simulink model "AGTF30SysDyn_PExPIn"  (R2023b)
settings: Solver=ode4  StartTime=0.0  StopTime=MWS.In.tend  FixedStep=MWS.In.Ts  RelTol=1e-3  EnableMultiTasking=on
model workspace: external: MAT-File (data not in the file)
values from neighbouring files (symbols this model uses):
  MWS = setup_initialize(MWS,startPt,SSsolverSP)    [Setup_Simulation.m]    (also in run_AGTF30e_script.m = Setup_Simulation(inputMethod,MWS.In,filename,Mdl,SSsolverSP))
undefined symbols (not defined in the file or in its folder): DiscIntNeverNeededParam
libraries: simulink x32, Lib_Solve_ModelSource_TMATS x28, Lib_EMTAT x27, Lib_Cntrl_FirstOrderSensor_TMATS x19, Lib_Cntrl_FirstOrderActuator_TMATS x2, Lib_Cntrl_LimitSelect_TMATS x2, Lib_Solve_OuterLoopIntegrator_TMATS x2, Lib_Cntrl_CorrectedSpeed_TMATS x1, Lib_Solve_IterNRSolverJC_TMATS x1, slpidlib x1
(part 5 of 8)

== system AGTF30SysDyn_PExPIn/Control System/Wf Controller/Controller/Wf Limit Controllers/Accel Controller ==
  Alt : Inport
  MN : Inport  Port=2
  N1cN : Inport  Port=3
  phiEPT : Inport  Port=4
  phiBoost : Inport  Port=5
  Wfmax : Inport  Port=6
  Wfcmd : Inport  Port=7
  ps3 : Inport  Port=8
  Constant : Constant  Value=MWS.In.Options.WfTransientLogic
  Constant1 : Constant  Value=MWS.In.Options.HybridConfig
  Constant10 : Constant  Value=MWS.In.Options.HybridConfig
  Constant11 : Constant  Value=1.0425
  Constant2 : Constant
  Constant3 : Constant  Value=-4*MWS.In.Ts
  Constant4 : Constant  Value=MWS.In.Options.TEEM
  Constant5 : Constant
  Constant6 : Constant  Value=1.068
  Constant7 : Constant  Value=1.04
  Constant8 : Constant  Value=MWS.In.Options.EngineEMInt
  Constant9 : Constant  Value=1.06
  Divide1 : Product  Inputs=**
  Divide2 : Product  Inputs=**
  Divide3 : Product  Inputs=*/
  Divide4 : Product  Inputs=**
  Gain2 : Gain  Gain=MWS.Cntrl.WfCntrl.GenAccel.CeilingMultiplier
  Math Function : Math
  Memory : Memory  InitialCondition=MWS.Init.IC.Wf
  Multiport Switch : MultiPortSwitch  SaturateOnIntegerOverflow=off  InputSameDT=off
  Multiport Switch1 : MultiPortSwitch  SaturateOnIntegerOverflow=off  InputSameDT=off
  RUSched_Boost : Lookup_n-D  NumberOfTableDimensions=5  BreakpointsForDimension1=MWS.Cntrl.WfCntrl.Accel.Boost.RUsch.N1cN_vec  BreakpointsForDimension2=MWS.Cntrl.WfCntrl.Accel.Boost.RUsch.Alt_vec  BreakpointsForDimension3=MWS.Cntrl.WfCntrl.Accel.Boost.RUsch.MN_vec  BreakpointsForDimension4=MWS.Cntrl.WfCntrl.Accel.Boost.RUsch.phiEPT_vec  BreakpointsForDimension5=MWS.Cntrl.WfCntrl.Accel.Boost.RUsch.phiBoost_vec  Table=MWS.Cntrl.WfCntrl.Accel.Boost.RUsch.RU_array  ExtrapMethod=Clip  InternalRulePriority=Speed  RndMeth=Simplest
      settings: InputPortMap=u0,u1,u2,u3,u4
  RUSched_PEx : Lookup_n-D  NumberOfTableDimensions=4  BreakpointsForDimension1=MWS.Cntrl.WfCntrl.Accel.PEx.RUsch.N1cN_vec  BreakpointsForDimension2=MWS.Cntrl.WfCntrl.Accel.PEx.RUsch.Alt_vec  BreakpointsForDimension3=MWS.Cntrl.WfCntrl.Accel.PEx.RUsch.MN_vec  BreakpointsForDimension4=MWS.Cntrl.WfCntrl.Accel.PEx.RUsch.phiEPT_vec  Table=MWS.Cntrl.WfCntrl.Accel.PEx.RUsch.RU_array  ExtrapMethod=Clip  InternalRulePriority=Speed  RndMeth=Simplest
      settings: InputPortMap=u0,u1,u2,u3
  RUSched_STD : Lookup_n-D  NumberOfTableDimensions=4  BreakpointsForDimension1=MWS.Cntrl.WfCntrl.Accel.STD.RUsch.N1cN_vec  BreakpointsForDimension2=MWS.Cntrl.WfCntrl.Accel.STD.RUsch.Alt_vec  BreakpointsForDimension3=MWS.Cntrl.WfCntrl.Accel.STD.RUsch.MN_vec  BreakpointsForDimension4=MWS.Cntrl.WfCntrl.Accel.STD.RUsch.phiEPT_vec  Table=MWS.Cntrl.WfCntrl.Accel.STD.RUsch.RU_array  ExtrapMethod=Clip  InternalRulePriority=Speed  RndMeth=Simplest
      settings: InputPortMap=u0,u1,u2,u3
  Settling Time Lookup : Lookup_n-D  NumberOfTableDimensions=1  BreakpointsForDimension1=MWS.Cntrl.WfCntrl.GenAccel.Alt_vec  BreakpointsForDimension2=MWS.Cntrl.STD.Wf.CntrlLimits.Cntrl.RUmax.Alt_vec  BreakpointsForDimension3=MWS.Cntrl.STD.Wf.CntrlLimits.Cntrl.RUmax.MN_vec  Table=MWS.Cntrl.WfCntrl.GenAccel.ts_vec  ExtrapMethod=Clip  InternalRulePriority=Speed  RndMeth=Simplest
  Sum : Sum  Inputs=|+-
  Sum1 : Sum  Inputs=|+-
  Sum2 : Sum  Inputs=|++
  Switch : Switch  Criteria=u2 > Threshold  Threshold=1.5  SaturateOnIntegerOverflow=off  InputSameDT=off
  Switch1 : Switch  Criteria=u2 > Threshold  Threshold=0.5  SaturateOnIntegerOverflow=off  InputSameDT=off
  Switch2 : Switch  Criteria=u2 > Threshold  Threshold=1.5  SaturateOnIntegerOverflow=off  InputSameDT=off
  Wfdmd : Outport  VectorParamsAs1DForOutWhenUnconnected=off
  WfmaxAccel_SP : Outport  Port=2  VectorParamsAs1DForOutWhenUnconnected=off
  wires:
  Gain2/1 -> Sum/1
  Divide2/1 -> Sum2/1
  Switch/1 -> Wfdmd/1, WfmaxAccel_SP/1
  Sum1/1 -> Divide2/1
  Divide3/1 -> Math Function/1
  Settling Time Lookup/1 -> Divide3/2
  Constant3/1 -> Divide3/1
  Alt/1 -> RUSched_Boost/2, RUSched_STD/2, RUSched_PEx/2, Settling Time Lookup/1
  Sum/1 -> Divide2/2
  Math Function/1 -> Sum1/2
  Constant2/1 -> Sum1/1
  Memory/1 -> Sum/2, Sum2/2
  Wfmax/1 -> Gain2/1
  Wfcmd/1 -> Memory/1
  Constant/1 -> Switch/2
  Sum2/1 -> Switch/3
  Constant1/1 -> Multiport Switch/1
  MN/1 -> RUSched_STD/3, RUSched_PEx/3, RUSched_Boost/3
  phiEPT/1 -> RUSched_STD/4, RUSched_PEx/4, RUSched_Boost/4
  phiBoost/1 -> RUSched_Boost/5
  RUSched_STD/1 -> Multiport Switch/2
  RUSched_Boost/1 -> Multiport Switch/3
  RUSched_PEx/1 -> Multiport Switch/4
  ps3/1 -> Divide1/2
  Multiport Switch/1 -> Divide4/2
  Divide1/1 -> Switch/1
  N1cN/1 -> RUSched_PEx/1, RUSched_Boost/1, RUSched_STD/1
  Divide4/1 -> Divide1/1
  Constant4/1 -> Switch1/2
  Constant6/1 -> Switch1/3
  Switch1/1 -> Divide4/1
  Constant8/1 -> Switch2/2
  Constant5/1 -> Switch2/3
  Switch2/1 -> Switch1/1
  Constant7/1 -> Multiport Switch1/2
  Constant9/1 -> Multiport Switch1/3
  Multiport Switch1/1 -> Switch2/1
  Constant10/1 -> Multiport Switch1/1
  Constant11/1 -> Multiport Switch1/4

== system AGTF30SysDyn_PExPIn/Control System/Wf Controller/Controller/Wf Limit Controllers/Decel Controller ==
  Alt : Inport
  MN : Inport  Port=2
  N1cN : Inport  Port=3
  phiEPT : Inport  Port=4
  phiBoost : Inport  Port=5
  Wfmin : Inport  Port=6
  Wf : Inport  Port=7
  ps3 : Inport  Port=8
  Compare To Constant : simulink/Logic and Bit Operations/Compare To Constant  relop=>=  const=1.5  OutDataTypeStr=boolean
  Compare To Constant1 : simulink/Logic and Bit Operations/Compare To Constant  relop=<=  const=0.1  OutDataTypeStr=boolean
  Constant : Constant  Value=MWS.In.Options.WfTransientLogic
  Constant1 : Constant  Value=MWS.In.Options.HybridConfig
  Constant2 : Constant
  Constant3 : Constant  Value=-4*MWS.In.Ts
  Constant4 : Constant  Value=MWS.In.Options.EngineEMInt
  Constant5 : Constant  Value=0.95
  Constant6 : Constant
  Constant7 : Constant  Value=0.94
  Divide1 : Product  Inputs=**
  Divide2 : Product  Inputs=**
  Divide3 : Product  Inputs=*/
  Divide4 : Product  Inputs=**
  Gain2 : Gain  Gain=MWS.Cntrl.WfCntrl.GenDecel.FloorMultiplier
  Logical Operator : Logic  AllPortsSameDT=off  OutDataTypeStr=boolean
  Math Function : Math
  Memory : Memory  InitialCondition=MWS.Init.IC.Wf
  Multiport Switch : MultiPortSwitch  SaturateOnIntegerOverflow=off  InputSameDT=off
  RUSched_Boost : Lookup_n-D  NumberOfTableDimensions=5  BreakpointsForDimension1=MWS.Cntrl.WfCntrl.Decel.Boost.RUsch.N1cN_vec  BreakpointsForDimension2=MWS.Cntrl.WfCntrl.Decel.Boost.RUsch.Alt_vec  BreakpointsForDimension3=MWS.Cntrl.WfCntrl.Decel.Boost.RUsch.MN_vec  BreakpointsForDimension4=MWS.Cntrl.WfCntrl.Decel.Boost.RUsch.phiEPT_vec  BreakpointsForDimension5=MWS.Cntrl.WfCntrl.Decel.Boost.RUsch.phiBoost_vec  Table=MWS.Cntrl.WfCntrl.Decel.Boost.RUsch.RU_array  ExtrapMethod=Clip  InternalRulePriority=Speed  RndMeth=Simplest
      settings: InputPortMap=u0,u1,u2,u3,u4
  RUSched_PEx : Lookup_n-D  NumberOfTableDimensions=4  BreakpointsForDimension1=MWS.Cntrl.WfCntrl.Decel.PEx.RUsch.N1cN_vec  BreakpointsForDimension2=MWS.Cntrl.WfCntrl.Decel.PEx.RUsch.Alt_vec  BreakpointsForDimension3=MWS.Cntrl.WfCntrl.Decel.PEx.RUsch.MN_vec  BreakpointsForDimension4=MWS.Cntrl.WfCntrl.Decel.PEx.RUsch.phiEPT_vec  Table=MWS.Cntrl.WfCntrl.Decel.PEx.RUsch.RU_array  ExtrapMethod=Clip  InternalRulePriority=Speed  RndMeth=Simplest
      settings: InputPortMap=u0,u1,u2,u3
  RUSched_STD : Lookup_n-D  NumberOfTableDimensions=4  BreakpointsForDimension1=MWS.Cntrl.WfCntrl.Decel.STD.RUsch.N1cN_vec  BreakpointsForDimension2=MWS.Cntrl.WfCntrl.Decel.STD.RUsch.Alt_vec  BreakpointsForDimension3=MWS.Cntrl.WfCntrl.Decel.STD.RUsch.MN_vec  BreakpointsForDimension4=MWS.Cntrl.WfCntrl.Decel.STD.RUsch.phiEPT_vec  Table=MWS.Cntrl.WfCntrl.Decel.STD.RUsch.RU_array  ExtrapMethod=Clip  InternalRulePriority=Speed  RndMeth=Simplest
      settings: InputPortMap=u0,u1,u2,u3
  Settling Time Lookup : Lookup_n-D  NumberOfTableDimensions=1  BreakpointsForDimension1=MWS.Cntrl.WfCntrl.GenDecel.Alt_vec  BreakpointsForDimension2=MWS.Cntrl.STD.Wf.CntrlLimits.Cntrl.RUmax.Alt_vec  BreakpointsForDimension3=MWS.Cntrl.STD.Wf.CntrlLimits.Cntrl.RUmax.MN_vec  Table=MWS.Cntrl.WfCntrl.GenDecel.ts_vec  ExtrapMethod=Clip  InternalRulePriority=Speed  RndMeth=Simplest
  Sum : Sum  Inputs=|+-
  Sum1 : Sum  Inputs=|+-
  Sum2 : Sum  Inputs=|++
  Switch : Switch  Criteria=u2 > Threshold  Threshold=1.5  SaturateOnIntegerOverflow=off  InputSameDT=off
  Switch1 : Switch  Criteria=u2 > Threshold  Threshold=0.5  SaturateOnIntegerOverflow=off  InputSameDT=off
  Switch2 : Switch  Criteria=u2 > Threshold  Threshold=1.5  SaturateOnIntegerOverflow=off  InputSameDT=off
  Wfdmd : Outport  VectorParamsAs1DForOutWhenUnconnected=off
  WfminDecel_SP : Outport  Port=2  VectorParamsAs1DForOutWhenUnconnected=off
  wires:
  Gain2/1 -> Sum/1
  Divide2/1 -> Sum2/1
  Sum/1 -> Divide2/2
  Constant2/1 -> Sum1/1
  Memory/1 -> Sum/2, Sum2/2
  Settling Time Lookup/1 -> Divide3/2
  Math Function/1 -> Sum1/2
  Divide3/1 -> Math Function/1
  Sum1/1 -> Divide2/1
  Constant3/1 -> Divide3/1
  Switch/1 -> WfminDecel_SP/1, Wfdmd/1
  Wf/1 -> Memory/1
  Wfmin/1 -> Gain2/1
  RUSched_PEx/1 -> Multiport Switch/4
  RUSched_STD/1 -> Multiport Switch/2
  Alt/1 -> RUSched_STD/2, RUSched_Boost/2, RUSched_PEx/2, Settling Time Lookup/1
  MN/1 -> RUSched_STD/3, RUSched_Boost/3, RUSched_PEx/3
  phiEPT/1 -> RUSched_Boost/4, RUSched_PEx/4, RUSched_STD/4
  phiBoost/1 -> RUSched_Boost/5
  Constant1/1 -> Switch2/2, Multiport Switch/1
  Constant/1 -> Switch/2
  RUSched_Boost/1 -> Multiport Switch/3
  Sum2/1 -> Switch/3
  ps3/1 -> Divide1/2
  Multiport Switch/1 -> Divide4/2
  Divide1/1 -> Switch/1
  N1cN/1 -> Compare To Constant1/1, RUSched_Boost/1, RUSched_PEx/1, RUSched_STD/1
  Constant6/1 -> Switch1/3
  Divide4/1 -> Divide1/1
  Switch1/1 -> Divide4/1
  Constant4/1 -> Compare To Constant/1
  Compare To Constant/1 -> Logical Operator/2
  Logical Operator/1 -> Switch1/2
  Compare To Constant1/1 -> Logical Operator/1
  Constant5/1 -> Switch2/3
  Constant7/1 -> Switch2/1
  Switch2/1 -> Switch1/1

== system AGTF30SysDyn_PExPIn/EngineSystem/Power System/Electrical Power System/EM Variant Subsystem/Scalar DEM Subsystem ==
  note: LPS
  note: HPS
  Vs [V] : Inport
  NemL [rpm] : Inport  Port=2
  TrqEML [ft-lb] : Inport  Port=3
  NemH [rpm] : Inport  Port=4
  TrqEMH [ft-lb] : Inport  Port=5
  Bus Selector18 : BusSelector  OutputSignals=P_2; W
  Bus Selector19 : BusSelector  OutputSignals=Pmech; W,Pelec; W
  Bus Selector20 : BusSelector  OutputSignals=P_DC; W
  Bus Selector21 : BusSelector  OutputSignals=P_2; W
  Bus Selector27 : BusSelector  OutputSignals=Pmech; W,Pelec; W
  Bus Selector28 : BusSelector  OutputSignals=P_DC; W
  Cable5 : Lib_EMTAT/Components/Power Flow/Cable  R=MWS.EPS.Cable.R
      settings: AttributesFormatString=Cable  SourceProductName=EMTAT
  Cable6 : Lib_EMTAT/Components/Power Flow/Cable  R=MWS.EPS.Cable.R
      settings: AttributesFormatString=Cable  SourceProductName=EMTAT
  Constant{57..58,60..63,67,69,71..72} (10 alike) : Constant  Value=0
  DC-AC Inverter (Efficiency Map) : Lib_EMTAT/Components/Power Flow/DC-AC Inverter (Efficiency Map)  X_C_VoltageInVec_M=MWS.EPS.InvL.Vvec  Y_C_RMSCurrentOutVec_M=MWS.EPS.InvL.Ivec  T_C_EffArray_M=MWS.EPS.InvL.Eff  K_e=MWS.EPS.InvL.K_emf  FM=0
      settings: AttributesFormatString=DC-AC Inverter (Efficiency Map)  SourceProductName=EMTAT
  DC-AC Inverter (Efficiency Map)1 : Lib_EMTAT/Components/Power Flow/DC-AC Inverter (Efficiency Map)  X_C_VoltageInVec_M=MWS.EPS.InvH.Vvec  Y_C_RMSCurrentOutVec_M=MWS.EPS.InvH.Ivec  T_C_EffArray_M=MWS.EPS.InvH.Eff  K_e=MWS.EPS.InvH.K_emf  FM=0
      settings: AttributesFormatString=DC-AC Inverter (Efficiency Map)  SourceProductName=EMTAT
  Mux2 : Mux  Inputs=[1 1 1 1 1]
  Mux3 : Mux  Inputs=[1 1 1 1 1]
  Mux6 : Mux  Inputs=2
  PCabqPEM Calc : Subsystem
  PCabqPEM Calc1 : Subsystem
  Terminator{14,16..18,24,38..40} (8 alike) : Terminator
  Three Phase Electric Machine (Sink)3 : Lib_EMTAT/Components/Power Flow/Three Phase Electric Machine (Sink)  X_C_SpeedVec_M=MWS.EPS.EML.Nvec  Y_C_TorqueVec_M=MWS.EPS.EML.Tvec  T_C_EffArray_M=MWS.EPS.EML.Eff  FM=0
      settings: SourceProductName=EMTAT
      settings: AttributesFormatString=|
      | Three Phase Electric Machine
      | (Sink)
  Three Phase Electric Machine (Sink)4 : Lib_EMTAT/Components/Power Flow/Three Phase Electric Machine (Sink)  X_C_SpeedVec_M=MWS.EPS.EMH.Nvec  Y_C_TorqueVec_M=MWS.EPS.EMH.Tvec  T_C_EffArray_M=MWS.EPS.EMH.Eff  FM=0
      settings: SourceProductName=EMTAT
      settings: AttributesFormatString=|
      | Three Phase Electric Machine
      | (Sink)
  Unit Delay : UnitDelay  InitialCondition=MWS.EPS.Cable.Iout_IC  SampleTime=-1  HasFrameUpgradeWarning=on
  Unit Delay1 : UnitDelay  InitialCondition=MWS.EPS.Cable.Iout_IC  SampleTime=-1  HasFrameUpgradeWarning=on
  W to hp : Gain  Gain=1/745.7
  W to hp4 : Gain  Gain=1/745.7
  Io [A] : Outport
  Out_LPEMbranch : Outport  Port=2
  Out_HPEMbranch : Outport  Port=3
  wires:
  Constant63/1 -> Cable5/3
  Bus Selector19/1 -> W to hp4/1  "<Pmech; W>"
  Three Phase Electric Machine (Sink)4/4 -> DC-AC Inverter (Efficiency Map)1/3
  Three Phase Electric Machine (Sink)4/2 -> Bus Selector19/1
  W to hp/1 -> [LPEMMotor_PwrMech]
  TrqEML [ft-lb]/1 -> Three Phase Electric Machine (Sink)3/3
  Unit Delay/1 -> Cable6/4
  Three Phase Electric Machine (Sink)3/4 -> DC-AC Inverter (Efficiency Map)/3
  Cable6/2 -> Bus Selector18/1
  Cable6/3 -> Terminator14/1
  DC-AC Inverter (Efficiency Map)1/1 -> Three Phase Electric Machine (Sink)4/1
  Unit Delay1/1 -> Cable5/4
  Three Phase Electric Machine (Sink)3/2 -> Bus Selector27/1
  Constant67/1 -> Three Phase Electric Machine (Sink)3/5
  DC-AC Inverter (Efficiency Map)/2 -> Bus Selector28/1
  Bus Selector27/2 -> [LPEMMotor_PwrElec]  "<Pelec; W>"
  Constant58/1 -> Three Phase Electric Machine (Sink)3/4
  Constant60/1 -> Three Phase Electric Machine (Sink)4/5
  Mux6/1 -> Io [A]/1
  Three Phase Electric Machine (Sink)3/3 -> Terminator38/1
  Cable6/1 -> DC-AC Inverter (Efficiency Map)/1
  TrqEMH [ft-lb]/1 -> Three Phase Electric Machine (Sink)4/3
  Cable5/3 -> Terminator24/1
  DC-AC Inverter (Efficiency Map)/4 -> Cable6/2
  Cable5/4 -> Mux6/2  "I_HPS [A]"
  Three Phase Electric Machine (Sink)3/1 -> Terminator39/1
  DC-AC Inverter (Efficiency Map)1/3 -> Terminator18/1
  Constant57/1 -> Three Phase Electric Machine (Sink)4/4
  Three Phase Electric Machine (Sink)4/3 -> Terminator16/1
  Cable5/1 -> DC-AC Inverter (Efficiency Map)1/1
  Constant62/1 -> DC-AC Inverter (Efficiency Map)1/5
  Constant69/1 -> Cable6/3
  Bus Selector20/1 -> [HPEMInvRect_Pwr]  "<P_DC; W>"
  Bus Selector28/1 -> [LPEMInvRect_Pwr]  "<P_DC; W>"
  Three Phase Electric Machine (Sink)4/1 -> Terminator17/1
  DC-AC Inverter (Efficiency Map)/1 -> Three Phase Electric Machine (Sink)3/1
  Cable5/2 -> Bus Selector21/1
  Constant71/1 -> DC-AC Inverter (Efficiency Map)/4
  Cable6/5 -> Unit Delay/1
  Cable5/5 -> Unit Delay1/1
  DC-AC Inverter (Efficiency Map)1/2 -> Bus Selector20/1
  Bus Selector21/1 -> [HPEMMotorCable_Pwr]  "<P_2; W>"
  DC-AC Inverter (Efficiency Map)/3 -> Terminator40/1
  Cable6/4 -> Mux6/1  "I_LPS [A]"
  Vs [V]/1 -> Cable6/1, Cable5/1
  W to hp4/1 -> [HPEMMotor_PwrMech]
  Bus Selector27/1 -> W to hp/1  "<Pmech; W>"
  Constant72/1 -> DC-AC Inverter (Efficiency Map)/5
  DC-AC Inverter (Efficiency Map)1/4 -> Cable5/2
  Bus Selector18/1 -> [LPEMMotorCable_Pwr]  "<P_2; W>"
  Constant61/1 -> DC-AC Inverter (Efficiency Map)1/4
  NemL [rpm]/1 -> DC-AC Inverter (Efficiency Map)/2, Three Phase Electric Machine (Sink)3/2
  NemH [rpm]/1 -> DC-AC Inverter (Efficiency Map)1/2, Three Phase Electric Machine (Sink)4/2
  [HPEMInvRect_Pwr] -> Mux3/3
  [HPEMMotor_PwrMech] -> Mux3/4
  [HPEMMotor_PwrElec] -> Mux3/2
  [LPEMInvRect_Pwr] -> Mux2/3
  [LPEMMotorCable_Pwr] -> Mux2/4
  [LPEMMotor_PwrElec] -> Mux2/2
  Mux3/1 -> Out_HPEMbranch/1
  [HPEMMotorCable_Pwr] -> Mux3/1
  [LPEMMotor_PwrMech] -> Mux2/1
  Mux2/1 -> Out_LPEMbranch/1
  Bus Selector19/2 -> [HPEMMotor_PwrElec]  "<Pelec; W>"
  [LPBranch_PCabqPEM] -> Mux2/5
  [HPBranch_PCabqPEM] -> Mux3/5
  [HPEMMotor_PwrMech] -> PCabqPEM Calc1/2(EMPwr)
  [HPEMMotorCable_Pwr] -> PCabqPEM Calc1/1(CablePwr)
  [LPEMMotorCable_Pwr] -> PCabqPEM Calc/1(CablePwr)
  [LPEMMotor_PwrMech] -> PCabqPEM Calc/2(EMPwr)
  PCabqPEM Calc/1(PCabqPEM) -> [LPBranch_PCabqPEM]
  PCabqPEM Calc1/1(PCabqPEM) -> [HPBranch_PCabqPEM]

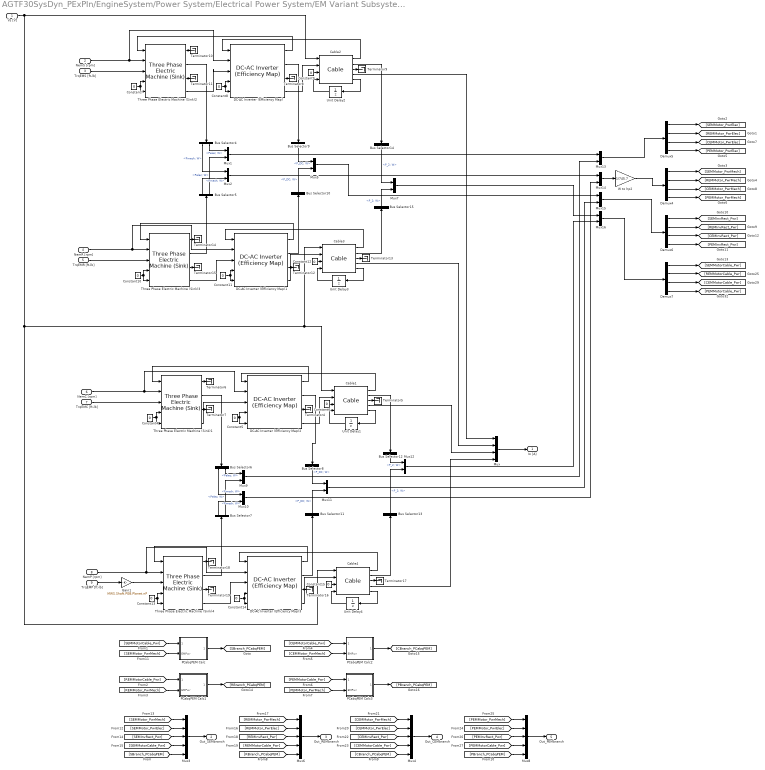
== system AGTF30SysDyn_PExPIn/EngineSystem/Power System/Electrical Power System/EM Variant Subsystem/Scalar PGB EM Subsystem ==
  Vs [V] : Inport
  NemS [rpm] : Inport  Port=2
  TrqEMS [ft-lb] : Inport  Port=3
  NemR [rpm] : Inport  Port=4
  TrqEMR [ft-lb] : Inport  Port=5
  NemC [rpm] : Inport  Port=6
  TrqEMC [ft-lb] : Inport  Port=7
  NemP [rpm] : Inport  Port=8
  TrqEMP [ft-lb] : Inport  Port=9
  Bus Selector{8..11} (4 alike) : BusSelector  OutputSignals=P_DC; W
  Bus Selector{12..15} (4 alike) : BusSelector  OutputSignals=P_2; W
  Bus Selector{4..7} (4 alike) : BusSelector  OutputSignals=Pmech; W,Pelec; W
  Cable{1..4} (4 alike) : Lib_EMTAT/Components/Power Flow/Cable  R=MWS.EPS.Cable.R
      settings: AttributesFormatString=Cable  SourceProductName=EMTAT
  Constant{4..15} (12 alike) : Constant  Value=0
  DC-AC Inverter (Efficiency Map) : Lib_EMTAT/Components/Power Flow/DC-AC Inverter (Efficiency Map)  X_C_VoltageInVec_M=MWS.EPS.InvS.Vvec  Y_C_RMSCurrentOutVec_M=MWS.EPS.InvS.Ivec  T_C_EffArray_M=MWS.EPS.InvS.Eff  K_e=MWS.EPS.InvS.K_emf  FM=0
      settings: AttributesFormatString=DC-AC Inverter (Efficiency Map)  SourceProductName=EMTAT
  DC-AC Inverter (Efficiency Map)1 : Lib_EMTAT/Components/Power Flow/DC-AC Inverter (Efficiency Map)  X_C_VoltageInVec_M=MWS.EPS.InvR.Vvec  Y_C_RMSCurrentOutVec_M=MWS.EPS.InvR.Ivec  T_C_EffArray_M=MWS.EPS.InvR.Eff  K_e=MWS.EPS.InvR.K_emf  FM=0
      settings: AttributesFormatString=DC-AC Inverter (Efficiency Map)  SourceProductName=EMTAT
  DC-AC Inverter (Efficiency Map)2 : Lib_EMTAT/Components/Power Flow/DC-AC Inverter (Efficiency Map)  X_C_VoltageInVec_M=MWS.EPS.InvC.Vvec  Y_C_RMSCurrentOutVec_M=MWS.EPS.InvC.Ivec  T_C_EffArray_M=MWS.EPS.InvC.Eff  K_e=MWS.EPS.InvC.K_emf  FM=0
      settings: AttributesFormatString=DC-AC Inverter (Efficiency Map)  SourceProductName=EMTAT
  DC-AC Inverter (Efficiency Map)3 : Lib_EMTAT/Components/Power Flow/DC-AC Inverter (Efficiency Map)  X_C_VoltageInVec_M=MWS.EPS.InvP.Vvec  Y_C_RMSCurrentOutVec_M=MWS.EPS.InvP.Ivec  T_C_EffArray_M=MWS.EPS.InvP.Eff  K_e=MWS.EPS.InvP.K_emf  FM=0
      settings: AttributesFormatString=DC-AC Inverter (Efficiency Map)  SourceProductName=EMTAT
  Demux{4..7} (4 alike) : Demux
  Gain1 : Gain  Gain=MWS.Shaft.PGB.Planet.nP
  Mux : Mux
  Mux{1..2,5,7,9..16} (12 alike) : Mux  Inputs=2
  Mux{3..4,6,8} (4 alike) : Mux  Inputs=[1 1 1 1 1]
  PCabqPEM Calc : Subsystem
  PCabqPEM Calc1 : Subsystem
  PCabqPEM Calc2 : Subsystem
  PCabqPEM Calc3 : Subsystem
  Terminator{4..19} (16 alike) : Terminator
  Three Phase Electric Machine (Sink)1 : Lib_EMTAT/Components/Power Flow/Three Phase Electric Machine (Sink)  X_C_SpeedVec_M=MWS.EPS.EMC.Nvec  Y_C_TorqueVec_M=MWS.EPS.EMC.Tvec  T_C_EffArray_M=MWS.EPS.EMC.Eff  FM=0
      settings: SourceProductName=EMTAT
      settings: AttributesFormatString=|
      | Three Phase Electric Machine
      | (Sink)
  Three Phase Electric Machine (Sink)2 : Lib_EMTAT/Components/Power Flow/Three Phase Electric Machine (Sink)  X_C_SpeedVec_M=MWS.EPS.EMS.Nvec  Y_C_TorqueVec_M=MWS.EPS.EMS.Tvec  T_C_EffArray_M=MWS.EPS.EMS.Eff  FM=0
      settings: SourceProductName=EMTAT
      settings: AttributesFormatString=|
      | Three Phase Electric Machine
      | (Sink)
  Three Phase Electric Machine (Sink)3 : Lib_EMTAT/Components/Power Flow/Three Phase Electric Machine (Sink)  X_C_SpeedVec_M=MWS.EPS.EMR.Nvec  Y_C_TorqueVec_M=MWS.EPS.EMR.Tvec  T_C_EffArray_M=MWS.EPS.EMR.Eff  FM=0
      settings: SourceProductName=EMTAT
      settings: AttributesFormatString=|
      | Three Phase Electric Machine
      | (Sink)
  Three Phase Electric Machine (Sink)4 : Lib_EMTAT/Components/Power Flow/Three Phase Electric Machine (Sink)  X_C_SpeedVec_M=MWS.EPS.EMP.Nvec  Y_C_TorqueVec_M=MWS.EPS.EMP.Tvec  T_C_EffArray_M=MWS.EPS.EMP.Eff  FM=0
      settings: SourceProductName=EMTAT
      settings: AttributesFormatString=|
      | Three Phase Electric Machine
      | (Sink)
  Unit Delay{1..4} (4 alike) : UnitDelay  InitialCondition=MWS.EPS.Cable.Iout_IC  SampleTime=-1  HasFrameUpgradeWarning=on
  W to hp2 : Gain  Gain=1/745.7
  Io [A] : Outport
  Out_SEMbranch : Outport  Port=2
  Out_REMbranch : Outport  Port=3
  Out_CEMbranch : Outport  Port=4
  Out_PEMbranch : Outport  Port=5
  wires:
  [PEMMotor_PwrElec] -> Mux8/2
  [SEMMotor_PwrMech] -> Mux3/1
  [PEMMotor_PwrMech] -> Mux8/1
  Mux3/1 -> Out_SEMbranch/1
  [REMMotor_PwrElec] -> Mux6/2
  Mux6/1 -> Out_REMbranch/1
  Mux8/1 -> Out_PEMbranch/1
  [SEMMotorCable_Pwr] -> Mux3/4
  [REMInvRect_Pwr] -> Mux6/3
  [REMMotor_PwrMech] -> Mux6/1
  [CEMInvRect_Pwr] -> Mux4/3
  [REMMotorCable_Pwr] -> Mux6/4
  [CEMMotor_PwrMech] -> Mux4/1
  [SEMMotor_PwrElec] -> Mux3/2
  [PEMInvRect_Pwr] -> Mux8/3
  [CEMMotor_PwrElec] -> Mux4/2
  Mux4/1 -> Out_CEMbranch/1
  [CEMMotorCable_Pwr] -> Mux4/4
  [SEMInvRect_Pwr] -> Mux3/3
  [PEMMotorCable_Pwr] -> Mux8/4
  TrqEMC [ft-lb]/1 -> Three Phase Electric Machine (Sink)1/3
  Three Phase Electric Machine (Sink)1/1 -> Terminator6/1
  Cable1/3 -> Terminator5/1
  DC-AC Inverter (Efficiency Map)2/1 -> Three Phase Electric Machine (Sink)1/1
  DC-AC Inverter (Efficiency Map)2/3 -> Terminator4/1
  Constant4/1 -> Three Phase Electric Machine (Sink)1/4, Three Phase Electric Machine (Sink)1/5
  Constant5/1 -> DC-AC Inverter (Efficiency Map)2/5, DC-AC Inverter (Efficiency Map)2/4
  Three Phase Electric Machine (Sink)1/4 -> DC-AC Inverter (Efficiency Map)2/3
  DC-AC Inverter (Efficiency Map)2/2 -> Bus Selector8/1
  Three Phase Electric Machine (Sink)1/2 -> Bus Selector6/1
  Cable1/4 -> Mux/3
  Cable1/1 -> DC-AC Inverter (Efficiency Map)2/1
  NemC [rpm]/1 -> DC-AC Inverter (Efficiency Map)2/2, Three Phase Electric Machine (Sink)1/2
  DC-AC Inverter (Efficiency Map)2/4 -> Cable1/2
  Three Phase Electric Machine (Sink)1/3 -> Terminator7/1
  Cable1/2 -> Bus Selector12/1
  Constant6/1 -> Cable1/3
  Unit Delay1/1 -> Cable1/4
  Cable1/5 -> Unit Delay1/1
  TrqEMS [ft-lb]/1 -> Three Phase Electric Machine (Sink)2/3
  Three Phase Electric Machine (Sink)2/1 -> Terminator10/1
  Cable2/3 -> Terminator9/1
  DC-AC Inverter (Efficiency Map)/1 -> Three Phase Electric Machine (Sink)2/1
  DC-AC Inverter (Efficiency Map)/3 -> Terminator8/1
  Constant7/1 -> Three Phase Electric Machine (Sink)2/4, Three Phase Electric Machine (Sink)2/5
  Constant8/1 -> DC-AC Inverter (Efficiency Map)/4, DC-AC Inverter (Efficiency Map)/5
  Three Phase Electric Machine (Sink)2/4 -> DC-AC Inverter (Efficiency Map)/3
  DC-AC Inverter (Efficiency Map)/2 -> Bus Selector9/1
  Three Phase Electric Machine (Sink)2/2 -> Bus Selector4/1
  Cable2/4 -> Mux/1
  Cable2/1 -> DC-AC Inverter (Efficiency Map)/1
  NemS [rpm]/1 -> DC-AC Inverter (Efficiency Map)/2, Three Phase Electric Machine (Sink)2/2
  DC-AC Inverter (Efficiency Map)/4 -> Cable2/2
  Three Phase Electric Machine (Sink)2/3 -> Terminator11/1
  Cable2/2 -> Bus Selector14/1
  Constant9/1 -> Cable2/3
  Unit Delay2/1 -> Cable2/4
  Cable2/5 -> Unit Delay2/1
  TrqEMR [ft-lb]/1 -> Three Phase Electric Machine (Sink)3/3
  Three Phase Electric Machine (Sink)3/1 -> Terminator14/1
  Cable3/3 -> Terminator13/1
  DC-AC Inverter (Efficiency Map)1/1 -> Three Phase Electric Machine (Sink)3/1
  DC-AC Inverter (Efficiency Map)1/3 -> Terminator12/1
  Constant10/1 -> Three Phase Electric Machine (Sink)3/4, Three Phase Electric Machine (Sink)3/5
  Constant11/1 -> DC-AC Inverter (Efficiency Map)1/4, DC-AC Inverter (Efficiency Map)1/5
  Three Phase Electric Machine (Sink)3/4 -> DC-AC Inverter (Efficiency Map)1/3
  DC-AC Inverter (Efficiency Map)1/2 -> Bus Selector10/1
  Three Phase Electric Machine (Sink)3/2 -> Bus Selector5/1
  Cable3/4 -> Mux/2
  Cable3/1 -> DC-AC Inverter (Efficiency Map)1/1
  NemR [rpm]/1 -> DC-AC Inverter (Efficiency Map)1/2, Three Phase Electric Machine (Sink)3/2
  DC-AC Inverter (Efficiency Map)1/4 -> Cable3/2
  Three Phase Electric Machine (Sink)3/3 -> Terminator15/1
  Cable3/2 -> Bus Selector15/1
  Constant12/1 -> Cable3/3
  Unit Delay3/1 -> Cable3/4
  Cable3/5 -> Unit Delay3/1
  DC-AC Inverter (Efficiency Map)3/2 -> Bus Selector11/1
  Cable4/2 -> Bus Selector13/1
  TrqEMP [ft-lb]/1 -> Gain1/1
  Unit Delay4/1 -> Cable4/4
  Constant15/1 -> Cable4/3
  DC-AC Inverter (Efficiency Map)3/4 -> Cable4/2
  Cable4/5 -> Unit Delay4/1
  Three Phase Electric Machine (Sink)4/3 -> Terminator19/1
  Cable4/1 -> DC-AC Inverter (Efficiency Map)3/1
  Cable4/4 -> Mux/4
  NemP [rpm]/1 -> DC-AC Inverter (Efficiency Map)3/2, Three Phase Electric Machine (Sink)4/2
  Three Phase Electric Machine (Sink)4/4 -> DC-AC Inverter (Efficiency Map)3/3
  Vs [V]/1 -> Cable1/1, Cable3/1, Cable4/1, Cable2/1
  Three Phase Electric Machine (Sink)4/1 -> Terminator18/1
  Constant14/1 -> DC-AC Inverter (Efficiency Map)3/4, DC-AC Inverter (Efficiency Map)3/5
  Constant13/1 -> Three Phase Electric Machine (Sink)4/4, Three Phase Electric Machine (Sink)4/5
  Cable4/3 -> Terminator17/1
  DC-AC Inverter (Efficiency Map)3/3 -> Terminator16/1
  DC-AC Inverter (Efficiency Map)3/1 -> Three Phase Electric Machine (Sink)4/1
  Three Phase Electric Machine (Sink)4/2 -> Bus Selector7/1
  Bus Selector4/2 -> Mux1/1  "<Pelec; W>"
  Bus Selector5/2 -> Mux1/2  "<Pelec; W>"
  Bus Selector4/1 -> Mux2/1  "<Pmech; W>"
  Bus Selector5/1 -> Mux2/2  "<Pmech; W>"
  Bus Selector9/1 -> Mux5/1  "<P_DC; W>"
  Bus Selector10/1 -> Mux5/2  "<P_DC; W>"
  Bus Selector14/1 -> Mux7/1  "<P_2; W>"
  Bus Selector15/1 -> Mux7/2  "<P_2; W>"
  Bus Selector7/2 -> Mux9/2  "<Pelec; W>"
  Bus Selector7/1 -> Mux10/2  "<Pmech; W>"
  Bus Selector6/1 -> Mux10/1  "<Pmech; W>"
  Bus Selector6/2 -> Mux9/1  "<Pelec; W>"
  Bus Selector11/1 -> Mux11/2  "<P_DC; W>"
  Bus Selector8/1 -> Mux11/1  "<P_DC; W>"
  Bus Selector13/1 -> Mux12/2  "<P_2; W>"
  Bus Selector12/1 -> Mux12/1  "<P_2; W>"
  Mux/1 -> Io [A]/1
  Mux1/1 -> Mux13/1
  Mux9/1 -> Mux13/2
  Mux10/1 -> Mux14/2
  Mux2/1 -> Mux14/1
  Mux12/1 -> Mux16/2
  Mux11/1 -> Mux15/2
  Mux7/1 -> Mux16/1
  Mux5/1 -> Mux15/1
  Mux14/1 -> W to hp2/1
  Demux6/2 -> [REMInvRect_Pwr]
  Demux6/3 -> [CEMInvRect_Pwr]
  Demux6/1 -> [SEMInvRect_Pwr]
  Demux6/4 -> [PEMInvRect_Pwr]
  Mux15/1 -> Demux6/1
  Demux7/1 -> [SEMMotorCable_Pwr]
  Demux7/4 -> [PEMMotorCable_Pwr]
  Demux7/3 -> [CEMMotorCable_Pwr]
  Demux7/2 -> [REMMotorCable_Pwr]
  Mux16/1 -> Demux7/1
  Gain1/1 -> Three Phase Electric Machine (Sink)4/3
  [SEMMotorCable_Pwr] -> PCabqPEM Calc/1(CablePwr)
  [SEMMotor_PwrMech] -> PCabqPEM Calc/2(EMPwr)
  [REMMotor_PwrMech] -> PCabqPEM Calc1/2(EMPwr)
  [REMMotorCable_Pwr] -> PCabqPEM Calc1/1(CablePwr)
  [PEMMotorCable_Pwr] -> PCabqPEM Calc3/1(CablePwr)
  [PEMMotor_PwrMech] -> PCabqPEM Calc3/2(EMPwr)
  [CEMMotor_PwrMech] -> PCabqPEM Calc2/2(EMPwr)
  [CEMMotorCable_Pwr] -> PCabqPEM Calc2/1(CablePwr)
  [SBranch_PCabqPEM] -> Mux3/5
  [RBranch_PCabqPEM] -> Mux6/5
  [CBranch_PCabqPEM] -> Mux4/5
  [PBranch_PCabqPEM] -> Mux8/5
  PCabqPEM Calc/1(PCabqPEM) -> [SBranch_PCabqPEM]
  PCabqPEM Calc1/1(PCabqPEM) -> [RBranch_PCabqPEM]
  PCabqPEM Calc2/1(PCabqPEM) -> [CBranch_PCabqPEM]
  PCabqPEM Calc3/1(PCabqPEM) -> [PBranch_PCabqPEM]
  Mux13/1 -> Demux5/1
  W to hp2/1 -> Demux4/1
  Demux4/1 -> [SEMMotor_PwrMech]
  Demux4/2 -> [REMMotor_PwrMech]
  Demux4/3 -> [CEMMotor_PwrMech]
  Demux4/4 -> [PEMMotor_PwrMech]
  Demux5/1 -> [SEMMotor_PwrElec]
  Demux5/2 -> [REMMotor_PwrElec]
  Demux5/3 -> [CEMMotor_PwrElec]
  Demux5/4 -> [PEMMotor_PwrElec]

== system AGTF30SysDyn_PExPIn/EngineSystem/Power System/Electrical Power System/Energy Storage Subsystem/DCDC Variant Subsystem ==
  V_ESD [V] : Inport
  I_Bus [A] : Inport  Port=2
  DCDC Regulator Subsystem : Subsystem  VariantControl=MWS.EPS.Options.DCDC == 0
  DCDC Set Point Subsystem : Subsystem  VariantControl=MWS.EPS.Options.DCDC == 1
  Io [A] : Outport
  Vo [V] : Outport  Port=2
  Outputs : Outport  Port=3

== system AGTF30SysDyn_PExPIn/EngineSystem/Power System/Electrical Power System/Energy Storage Subsystem/ESD Variant Subsystem ==
  I [A] : Inport
  ESD Battery Subsystem : Subsystem  VariantControl=MWS.EPS.Options.ESD == 0
  ESD Supercapacitor Subsystem : Subsystem  VariantControl=MWS.EPS.Options.ESD == 1
  Vo [V] : Outport
  SoC [%] : Outport  Port=2

== system AGTF30SysDyn_PExPIn/Control System/Electric Machine Controllers/EM Controllers/DEM Control/DEM EM Controllers/EMH Controller ==
  PwrInHPEMNomMan : Inport
  PwrInHPEMNomManEn : Inport  Port=2
  PwrInHPEMOffNomMan : Inport  Port=3
  PwrInHPEMOffNomManEn : Inport  Port=4
  PwrInHP_Base : Inport  Port=5
  NemH : Inport  Port=6
  PwrInHPEPT : Inport  Port=7
  PwrInAccel_TEEM : Inport  Port=8
  PwrXDecel_TEEM : Inport  Port=9
  PwrCharge : Inport  Port=10
  PwrSys : Inport  Port=11
  PExAC : Inport  Port=12
  Bus Selector1 : BusSelector  OutputSignals=Pwrs.EMHbranch
  Constant : Constant  Value=MWS.In.Options.HybridConfig
  Demux : Demux  Outputs=[4 1]
  Divide : Product  Inputs=*/
  Divide1 : Product  Inputs=**
  Divide2 : Product  Inputs=**
  Gain : Gain  Gain=5252.113
  Gain1 : Gain  Gain=1/5252.113
  Gain4 : Gain  Gain=-1
  Math Function : Math  Operator=reciprocal
  Memory : Memory  InitialCondition=1
  MinMax : MinMax
  Multiport Switch1 : MultiPortSwitch  SaturateOnIntegerOverflow=off  InputSameDT=off
  Mux : Mux  Inputs=2
  Pwr Saturation : Saturate  UpperLimit=MWS.PowerSystem.EMH.PMax  LowerLimit=-MWS.PowerSystem.EMH.PMax
  Sum{,1..2,4} (4 alike) : Sum  Inputs=|++
  Sum of Elements : Sum  Inputs=+
  Sum3 : Sum  Inputs=|+-
  Sum5 : Sum  Inputs=|+-
  Switch : Switch  Criteria=u2 > Threshold  SaturateOnIntegerOverflow=off  InputSameDT=off
  Switch1 : Switch  Criteria=u2 > Threshold  SaturateOnIntegerOverflow=off  InputSameDT=off
  Terminator : Terminator
  Trq Saturation : Saturate  UpperLimit=MWS.PowerSystem.EMH.TrqMax  LowerLimit=-MWS.PowerSystem.EMH.TrqMax
  PwrEMH : Outport
  TrqEMH : Outport  Port=2
  PwrLoadEMH : Outport  Port=3
  wires:
  Gain1/1 -> PwrEMH/1
  Divide1/1 -> Gain1/1
  Trq Saturation/1 -> Divide1/1, TrqEMH/1
  Divide/1 -> Trq Saturation/1
  NemH/1 -> Divide/2, Divide1/2
  Gain/1 -> Divide/1
  Pwr Saturation/1 -> Gain/1
  Sum/1 -> Pwr Saturation/1
  Sum1/1 -> Sum3/1  "Pwr_TEEM"
  PwrInHPEMOffNomMan/1 -> Switch1/1
  PwrInHPEMOffNomManEn/1 -> Switch1/2
  Switch1/1 -> Sum/2
  Switch/1 -> Sum/1
  PwrInHP_Base/1 -> [PwrInHP_Base], Sum2/1
  PwrInHPEMNomMan/1 -> Switch/1
  PwrInHPEMNomManEn/1 -> Switch/2
  PwrXDecel_TEEM/1 -> Sum1/2
  Sum2/1 -> Switch/3  "PwrSS"
  PwrInHPEPT/1 -> Sum2/2
  Sum3/1 -> Switch1/3  "Pwr_OffNom"
  PwrCharge/1 -> Sum3/2
  PwrInAccel_TEEM/1 -> Sum1/1
  MinMax/1 -> Memory/1
  [Eff] -> Divide2/2
  Sum of Elements/1 -> Gain4/1
  Multiport Switch1/1 -> Sum of Elements/1
  Gain4/1 -> PwrLoadEMH/1
  Constant/1 -> Multiport Switch1/1
  PwrSys/1 -> Bus Selector1/1
  [PwrInHP_Base] -> Sum4/1, Multiport Switch1/2, Multiport Switch1/3
  Math Function/1 -> Mux/2
  Bus Selector1/1 -> Demux/1  "<EMHbranch>"
  Demux/2 -> Mux/1, Math Function/1  "PCabqPEM"
  Demux/1 -> Terminator/1
  Memory/1 -> [Eff]
  Mux/1 -> MinMax/1
  PExAC/1 -> Sum5/2, Sum4/2
  Sum4/1 -> Divide2/1
  Divide2/1 -> Sum5/1
  Sum5/1 -> Multiport Switch1/4

== system AGTF30SysDyn_PExPIn/Control System/Electric Machine Controllers/EM Controllers/DEM Control/DEM EM Controllers/EML Controller ==
  PwrInLPEMNomMan : Inport
  PwrInLPEMNomManEn : Inport  Port=2
  PwrInLPEMOffNomMan : Inport  Port=3
  PwrInLPEMOffNomManEn : Inport  Port=4
  PwrInLP_Base : Inport  Port=5
  NemL : Inport  Port=6
  PwrInLPEPT : Inport  Port=7
  PwrExAccel_TEEM : Inport  Port=8
  PwrXDecel_TEEM : Inport  Port=9
  PwrSys : Inport  Port=10
  Bus Selector1 : BusSelector  OutputSignals=Pwrs.EMLbranch
  Constant : Constant  Value=MWS.In.Options.HybridConfig
  Constant1 : Constant  Value=0
  Constant2 : Constant  Value=0
  Demux : Demux  Outputs=[4 1]
  Divide : Product  Inputs=*/
  Divide1 : Product  Inputs=**
  Divide2 : Product  Inputs=**
  Gain : Gain  Gain=5252.113
  Gain1 : Gain  Gain=1/5252.113
  Gain2 : Gain  Gain=-1
  Gain3 : Gain  Gain=-1
  Gain4 : Gain  Gain=-1
  Math Function : Math  Operator=reciprocal
  Memory : Memory  InitialCondition=1
  MinMax : MinMax
  Multiport Switch1 : MultiPortSwitch  SaturateOnIntegerOverflow=off  InputSameDT=off
  Mux : Mux  Inputs=2
  Pwr Saturation : Saturate  UpperLimit=MWS.PowerSystem.EML.PMax  LowerLimit=-MWS.PowerSystem.EML.PMax
  Sum : Sum  Inputs=|++
  Sum of Elements : Sum  Inputs=+
  Sum1 : Sum  Inputs=|++
  Sum2 : Sum  Inputs=|++
  Switch : Switch  Criteria=u2 > Threshold  SaturateOnIntegerOverflow=off  InputSameDT=off
  Switch1 : Switch  Criteria=u2 > Threshold  SaturateOnIntegerOverflow=off  InputSameDT=off
  Terminator : Terminator
  Trq Saturation : Saturate  UpperLimit=MWS.PowerSystem.EML.TrqMax  LowerLimit=-MWS.PowerSystem.EML.TrqMax
  PwrEML : Outport
  TrqEML : Outport  Port=2
  PwrLoadL : Outport  Port=3
  wires:
  PwrInLPEMNomManEn/1 -> Switch/2
  PwrInLPEMNomMan/1 -> Switch/1
  PwrInLP_Base/1 -> [PwrInLP_Base], Sum1/1
  Switch/1 -> Sum/1
  Switch1/1 -> Sum/2
  PwrInLPEMOffNomManEn/1 -> Switch1/2
  PwrInLPEMOffNomMan/1 -> Switch1/1
  Gain2/1 -> Sum2/2  "PwrInLPS_TEEM"
  Sum/1 -> Pwr Saturation/1
  Pwr Saturation/1 -> Gain/1
  Gain/1 -> Divide/1
  NemL/1 -> Divide1/2, Divide/2
  Divide/1 -> Trq Saturation/1
  Trq Saturation/1 -> TrqEML/1, Divide1/1
  Divide1/1 -> Gain1/1
  Gain1/1 -> PwrEML/1
  PwrXDecel_TEEM/1 -> Gain2/1
  PwrInLPEPT/1 -> Sum1/2
  Sum1/1 -> Switch/3
  PwrExAccel_TEEM/1 -> Gain3/1
  Gain3/1 -> Sum2/1  "PwrInLPS_TEEM"
  Sum2/1 -> Switch1/3
  Sum of Elements/1 -> Gain4/1
  Gain4/1 -> PwrLoadL/1
  Constant/1 -> Multiport Switch1/1
  Multiport Switch1/1 -> Sum of Elements/1
  Constant1/1 -> Multiport Switch1/2
  Constant2/1 -> Multiport Switch1/3
  PwrSys/1 -> Bus Selector1/1
  Demux/1 -> Terminator/1
  Bus Selector1/1 -> Demux/1  "<EMLbranch>"
  Demux/2 -> Mux/1, Math Function/1  "PCabqPEM"
  [PwrInLP_Base] -> Divide2/1
  [Eff] -> Divide2/2
  Divide2/1 -> Multiport Switch1/4
  Math Function/1 -> Mux/2
  Mux/1 -> MinMax/1
  MinMax/1 -> Memory/1
  Memory/1 -> [Eff]

== system AGTF30SysDyn_PExPIn/Control System/Electric Machine Controllers/EM Controllers/DEM Control/DEM EM Controllers/EPT Pwr Calc ==
  PwrEPT : Inport
  Gain : Gain  Gain=-1
  PwrEML_EPT : Outport
  PwrEMH_EPT : Outport  Port=2
  wires:
  Gain/1 -> PwrEML_EPT/1
  PwrEPT/1 -> PwrEMH_EPT/1, Gain/1

== system AGTF30SysDyn_PExPIn/Control System/Electric Machine Controllers/EM Controllers/PGB EM Control/VEATE EM Controllers/Base Power ==
  note: STRATEGY WILL USE THE COUPLING EM AS MUCH AS POSSIBLE AND WILL FILL IN THE REST WITH THE OTHER EMs
      |
      | CHARGING POWER IS DERIVED FROM THE HP BECAUSE ALL CONFIGURATIONS SHOULD HAVE AN HP EM. IT WILL EFFECTIVELY RAISE THE SUBSYSTEM LOAD.
  note: OUTPUTS
  note: INPUTS
  note: BASE POWER CALCULATION
  note: Standard/Regular
      | Boost
      | Power Extraction
  PwrInLP_Base : Inport
  PwrInHP_Base : Inport  Port=2
  NS : Inport  Port=3
  NR : Inport  Port=4
  NC : Inport  Port=5
  PExAC : Inport  Port=6
  PwrSys : Inport  Port=7
  Base Power - Boost and PEx : Subsystem
  Base Power - Standard : Subsystem
  Constant2 : Constant  Value=MWS.In.Options.HybridConfig
  Demux2 : Demux
  Gain1 : Gain  Gain=-1
  Load Calc : Subsystem
  Multiport Switch : MultiPortSwitch  SaturateOnIntegerOverflow=off  InputSameDT=off
  Multiport Switch1 : MultiPortSwitch  SaturateOnIntegerOverflow=off  InputSameDT=off
  Sum of Elements1 : Sum  Inputs=+
  PwrEMS_Base : Outport
  PwrEMR_Base : Outport  Port=2
  PwrEMC_Base : Outport  Port=3
  PwrEMP_Base : Outport  Port=4
  PwrLoad : Outport  Port=5
  wires:
  PwrInLP_Base/1 -> [PwrL_Base]
  NR/1 -> [NR]
  NS/1 -> [NS]
  NC/1 -> [NC]
  PwrInHP_Base/1 -> [PwrH_Base]
  [PwrEMS_Base] -> PwrEMS_Base/1
  [PwrEMR_Base] -> PwrEMR_Base/1
  [PwrEMC_Base] -> PwrEMC_Base/1
  [PwrEMP_Base] -> PwrEMP_Base/1
  Constant2/1 -> Multiport Switch1/1, Multiport Switch/1
  Multiport Switch/1 -> Demux2/1
  Demux2/1 -> [PwrEMS_Base]
  Demux2/2 -> [PwrEMR_Base]
  Demux2/3 -> [PwrEMC_Base]
  Demux2/4 -> [PwrEMP_Base]
  [PwrH_Base] -> Base Power - Boost and PEx/2(PwrH_Base)
  [NS] -> Base Power - Boost and PEx/3(NS)
  [NR] -> Base Power - Boost and PEx/4(NR)
  [NC] -> Base Power - Boost and PEx/5(NC)
  Base Power - Boost and PEx/1(Pem) -> [Pem_BoostPEx]
  Base Power - Standard/1(Pem) -> [Pem_Std]
  [NC] -> Base Power - Standard/4(NC)
  [NR] -> Base Power - Standard/3(NR)
  [NS] -> Base Power - Standard/2(NS)
  [PwrH_Base] -> Base Power - Standard/1(PwrH_Base)
  [Pem_Std] -> Multiport Switch/2, Sum of Elements1/1
  [Pem_BoostPEx] -> Load Calc/1(PemBoost_PEx), Multiport Switch/4, Multiport Switch/3
  [PwrL_Base] -> Base Power - Boost and PEx/1(PwrL_Base)
  Multiport Switch1/1 -> [PwrLoad]
  [PwrLoad] -> PwrLoad/1
  Load Calc/1(PwrLoad) -> Multiport Switch1/4
  PExAC/1 -> [PExAC]
  [PExAC] -> Load Calc/2(PExAC)
  PwrSys/1 -> [PwrSys]
  [PwrSys] -> Load Calc/3(PwrSys)
  Sum of Elements1/1 -> Gain1/1
  Gain1/1 -> Multiport Switch1/2, Multiport Switch1/3

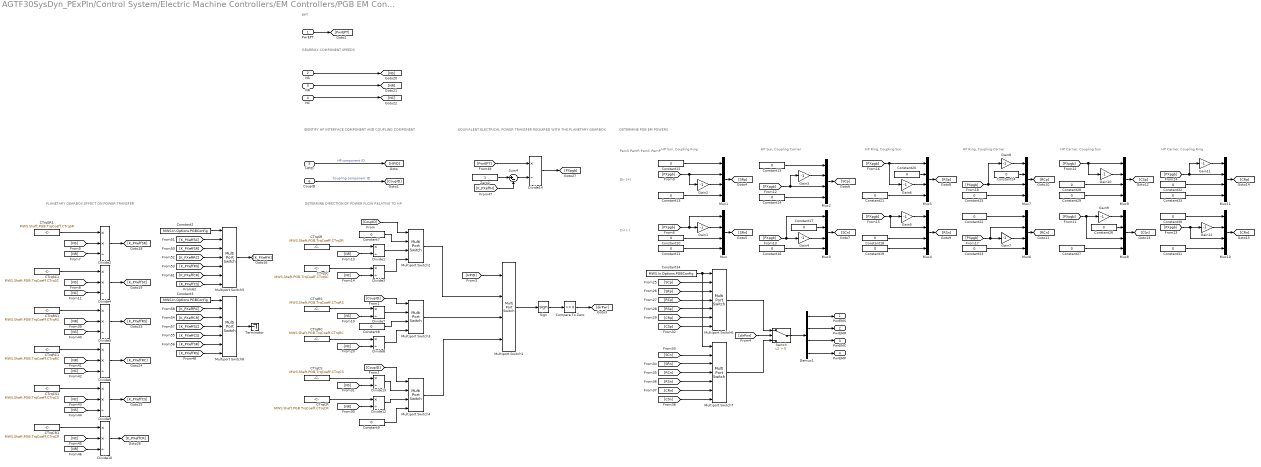
== system AGTF30SysDyn_PExPIn/Control System/Electric Machine Controllers/EM Controllers/PGB EM Control/VEATE EM Controllers/EPT Powers ==
  note: Dir (+)
  note: HP Sun, Coupling Ring
  note: PemS
      | PemR
      | PemC
      | PemP
  note: IDENTIFY HP INTERFACE COMPONENT AND COUPLING COMPONENT
  note: HP Sun, Coupling Carrier
  note: Dir (-)
  note: HP Ring, Coupling Sun
  note: HP Ring, Coupling Carrier
  note: HP Carrier, Coupling Sun
  note: HP Carrier, Coupling Ring
  note: DETERMINE DIRECTION OF POWER FLOW RELATIVE TO HP
  note: DETERMINE PGB EM POWERS
  note: GEARBOX COMPONENT SPEEDS
  note: EPT
  note: PLANETARY GEARBOX EFFECT ON POWER TRANSFER
  note: EQUIVALENT ELECTRICAL POWER TRANSFER REQUIRED WITH THE PLANETARY GEARBOX
  PwrEPT : Inport
  NS : Inport  Port=2
  NR : Inport  Port=3
  NC : Inport  Port=4
  HPID : Inport  Port=5
  CoupID : Inport  Port=6
  CTrqCR : Constant  Value=MWS.Shaft.PGB.TrqCoeff.CTrqCR
  CTrqCR1 : Constant  Value=MWS.Shaft.PGB.TrqCoeff.CTrqCR
  CTrqCS : Constant  Value=MWS.Shaft.PGB.TrqCoeff.CTrqCS
  CTrqCS1 : Constant  Value=MWS.Shaft.PGB.TrqCoeff.CTrqCS
  CTrqRC : Constant  Value=MWS.Shaft.PGB.TrqCoeff.CTrqRC
  CTrqRC1 : Constant  Value=MWS.Shaft.PGB.TrqCoeff.CTrqRC
  CTrqRS : Constant  Value=MWS.Shaft.PGB.TrqCoeff.CTrqRS
  CTrqRS1 : Constant  Value=MWS.Shaft.PGB.TrqCoeff.CTrqRS
  CTrqSC : Constant  Value=MWS.Shaft.PGB.TrqCoeff.CTrqSC
  CTrqSC1 : Constant  Value=MWS.Shaft.PGB.TrqCoeff.CTrqSC
  CTrqSR : Constant  Value=MWS.Shaft.PGB.TrqCoeff.CTrqSR
  CTrqSR1 : Constant  Value=MWS.Shaft.PGB.TrqCoeff.CTrqSR
  Compare To Zero : simulink/Logic and Bit Operations/Compare To Zero  relop=>=  OutDataTypeStr=boolean
  Constant{7..33} (27 alike) : Constant  Value=0
  Constant2 : Constant  Value=MWS.In.Options.PGBConfig
  Constant3 : Constant  Value=MWS.In.Options.PGBConfig
  Constant34 : Constant  Value=MWS.In.Options.PGBConfig
  Demux1 : Demux
  Divide{1,3,7..8,12..14} (7 alike) : Product  Inputs=*/
  Divide{2,4..6,9..10} (6 alike) : Product  Inputs=**/
  Gain{1..12} (12 alike) : Gain  Gain=-1
  Multiport Switch1 : MultiPortSwitch  SaturateOnIntegerOverflow=off  InputSameDT=off
  Multiport Switch2 : MultiPortSwitch  DataPortOrder=Specify indices  SaturateOnIntegerOverflow=off  InputSameDT=off
  Multiport Switch3 : MultiPortSwitch  DataPortOrder=Specify indices  SaturateOnIntegerOverflow=off  InputSameDT=off
  Multiport Switch4 : MultiPortSwitch  DataPortOrder=Specify indices  SaturateOnIntegerOverflow=off  InputSameDT=off
  Multiport Switch{5..8} (4 alike) : MultiPortSwitch  Inputs=6  SaturateOnIntegerOverflow=off  InputSameDT=off
  Mux{,1..11} (12 alike) : Mux
  Sign : Signum
  Sum4 : Sum  Inputs=|+-
  Switch : Switch  Criteria=u2 > Threshold  SaturateOnIntegerOverflow=off  InputSameDT=off
  Terminator : Terminator
  Zero2 : Constant
  PwrEMS : Outport
  PwrEMR : Outport  Port=2
  PwrEMC : Outport  Port=3
  PwrEMP : Outport  Port=4
  wires:
  HPID/1 -> [HPID]  "HP component ID"
  CoupID/1 -> [CoupID]  "Coupling component ID"
  CTrqSC/1 -> Divide3/1
  [NS] -> Divide13/2
  [NS] -> Divide7/2
  [NC] -> Divide8/2
  [NC] -> Divide3/2
  CTrqCR/1 -> Divide12/1
  [NR] -> Divide12/2
  [NR] -> Divide1/2
  CTrqCS/1 -> Divide13/1
  CTrqRS/1 -> Divide7/1
  CTrqRC/1 -> Divide8/1
  CTrqSR/1 -> Divide1/1
  Divide1/1 -> Multiport Switch2/3
  Divide3/1 -> Multiport Switch2/4
  Constant7/1 -> Multiport Switch2/2
  [CoupID] -> Multiport Switch2/1
  Divide7/1 -> Multiport Switch3/2
  Divide8/1 -> Multiport Switch3/4
  [CoupID] -> Multiport Switch3/1
  Constant8/1 -> Multiport Switch3/3
  Constant9/1 -> Multiport Switch4/4
  [CoupID] -> Multiport Switch4/1
  Divide13/1 -> Multiport Switch4/2
  Divide12/1 -> Multiport Switch4/3
  Multiport Switch3/1 -> Multiport Switch1/3
  Multiport Switch2/1 -> Multiport Switch1/2
  Multiport Switch4/1 -> Multiport Switch1/4
  [HPID] -> Multiport Switch1/1
  Multiport Switch1/1 -> Sign/1
  Sign/1 -> Compare To Zero/1
  Compare To Zero/1 -> [dirPwr]
  Gain1/1 -> Mux/2
  [PXpgb] -> Mux/1, Gain1/1
  Constant10/1 -> Mux/3
  Constant11/1 -> Mux/4
  Constant13/1 -> Mux1/4
  Constant12/1 -> Mux1/1
  [PXpgb] -> Mux1/2, Gain2/1
  Gain2/1 -> Mux1/3
  Constant14/1 -> Mux2/4
  [PXpgb] -> Mux2/3, Gain3/1
  Gain3/1 -> Mux2/2
  Constant15/1 -> Mux2/1
  [PXpgb] -> Mux3/1, Gain4/1
  Constant16/1 -> Mux3/4
  Gain4/1 -> Mux3/3
  Constant17/1 -> Mux3/2
  [PXpgb] -> Mux5/1, Gain6/1
  Constant19/1 -> Mux4/4
  [PXpgb] -> Mux4/2, Gain5/1
  Constant21/1 -> Mux5/4
  Gain6/1 -> Mux5/3
  Gain5/1 -> Mux4/1
  Constant20/1 -> Mux5/2
  Constant18/1 -> Mux4/3
  Constant24/1 -> Mux7/2
  Constant25/1 -> Mux7/4
  [PXpgb] -> Mux6/2, Gain7/1
  Constant23/1 -> Mux6/4
  [PXpgb] -> Mux7/3, Gain8/1
  Gain8/1 -> Mux7/1
  Gain7/1 -> Mux6/3
  Constant22/1 -> Mux6/1
  Gain9/1 -> Mux8/1
  Constant27/1 -> Mux8/4
  [PXpgb] -> Mux8/3, Gain9/1
  Gain10/1 -> Mux9/2
  Constant29/1 -> Mux9/4
  Constant26/1 -> Mux8/2
  [PXpgb] -> Gain10/1, Mux9/1
  Constant28/1 -> Mux9/3
  Constant32/1 -> Mux11/3
  [PXpgb] -> Mux11/2, Gain11/1
  Constant33/1 -> Mux11/4
  [PXpgb] -> Mux10/3, Gain12/1
  Constant31/1 -> Mux10/4
  Gain11/1 -> Mux11/1
  Gain12/1 -> Mux10/2
  Constant30/1 -> Mux10/1
  Mux1/1 -> [SRp]
  Mux/1 -> [SRn]
  Mux2/1 -> [SCp]
  Mux3/1 -> [SCn]
  Mux5/1 -> [RSp]
  Mux4/1 -> [RSn]
  Mux7/1 -> [RCp]
  Mux6/1 -> [RCn]
  Mux9/1 -> [CSp]
  Mux8/1 -> [CSn]
  Mux11/1 -> [CRp]
  Mux10/1 -> [CRn]
  [SCp] -> Multiport Switch6/2
  [SRp] -> Multiport Switch6/3
  [RCp] -> Multiport Switch6/4
  [RSp] -> Multiport Switch6/5
  [CRp] -> Multiport Switch6/6
  [CSp] -> Multiport Switch6/7
  [CSn] -> Multiport Switch7/7
  [CRn] -> Multiport Switch7/6
  [RSn] -> Multiport Switch7/5
  [RCn] -> Multiport Switch7/4
  [SRn] -> Multiport Switch7/3
  [SCn] -> Multiport Switch7/2
  Multiport Switch6/1 -> Switch/1
  Multiport Switch7/1 -> Switch/3
  Switch/1 -> Demux1/1
  Constant34/1 -> Multiport Switch7/1, Multiport Switch6/1
  Demux1/1 -> PwrEMS/1
  Demux1/2 -> PwrEMR/1
  Demux1/3 -> PwrEMC/1
  Demux1/4 -> PwrEMP/1
  PwrEPT/1 -> [PwrEPT]
  NS/1 -> [NS]
  NR/1 -> [NR]
  NC/1 -> [NC]
  [dirPwr] -> Switch/2
  CTrqSR1/1 -> Divide2/1
  [NR] -> Divide2/3
  [NS] -> Divide2/2
  CTrqSC1/1 -> Divide4/1
  [NS] -> Divide4/2
  [NC] -> Divide4/3
  CTrqRS1/1 -> Divide5/1
  [NR] -> Divide5/2
  [NS] -> Divide5/3
  CTrqRC1/1 -> Divide6/1
  [NR] -> Divide6/2
  [NC] -> Divide6/3
  CTrqCS1/1 -> Divide9/1
  [NC] -> Divide9/2
  [NS] -> Divide9/3
  CTrqCR1/1 -> Divide10/1
  [NC] -> Divide10/2
  [NR] -> Divide10/3
  Divide2/1 -> [K_PXeffSR]
  Divide4/1 -> [K_PXeffSC]
  Divide5/1 -> [K_PXeffRS]
  Divide6/1 -> [K_PXeffRC]
  Divide9/1 -> [K_PXeffCS]
  Divide10/1 -> [K_PXeffCR]
  [K_PXeffH] -> Sum4/2
  [PwrEPT] -> Divide14/1
  Sum4/1 -> Divide14/2
  Zero2/1 -> Sum4/1
  Constant2/1 -> Multiport Switch5/1
  [K_PXeffCS] -> Multiport Switch5/7
  [K_PXeffCR] -> Multiport Switch5/6
  [K_PXeffRS] -> Multiport Switch5/5
  [K_PXeffRC] -> Multiport Switch5/4
  [K_PXeffSR] -> Multiport Switch5/3
  [K_PXeffSC] -> Multiport Switch5/2
  Multiport Switch5/1 -> [K_PXeffH]
  Divide14/1 -> [PXpgb]
  [K_PXeffRC] -> Multiport Switch8/2
  Constant3/1 -> Multiport Switch8/1
  [K_PXeffCS] -> Multiport Switch8/5
  [K_PXeffRS] -> Multiport Switch8/7
  [K_PXeffCR] -> Multiport Switch8/3
  Multiport Switch8/1 -> Terminator/1
  [K_PXeffSC] -> Multiport Switch8/4
  [K_PXeffSR] -> Multiport Switch8/6

== system AGTF30SysDyn_PExPIn/Control System/Electric Machine Controllers/EM Controllers/PGB EM Control/VEATE EM Controllers/TEEM Power ==
  note: TEEM POWER CALCULATION
  note: INPUTS
  note: OUTPUTS
  note: STRATEGY WILL USE THE COUPLING EM AS MUCH AS POSSIBLE AND WILL FILL IN THE REST WITH THE OTHER EMs. OBJECTIVE IS TO ACHIEVE THE DESIRED HP POWER INPUT.
  PwrInHP_TEEM : Inport
  PwrExLP_TEEM : Inport  Port=2
  PwrInX_TEEM : Inport  Port=3
  NS : Inport  Port=4
  NR : Inport  Port=5
  NC : Inport  Port=6
  N1cErrN : Inport  Port=7
  Constant1 : Constant  Value=[0 0 0 0]
  Constant2 : Constant  Value=MWS.In.Options.TEEM
  Demux2 : Demux
  Switch : Switch  Criteria=u2 > Threshold  SaturateOnIntegerOverflow=off  InputSameDT=off
  TEEM Power : Subsystem
  PwrEMS_TEEM : Outport
  PwrEMR_TEEM : Outport  Port=2
  PwrEMC_TEEM : Outport  Port=3
  PwrEMP_TEEM : Outport  Port=4
  wires:
  TEEM Power/1(Pem) -> [Pem_TEEM]
  [NC] -> TEEM Power/6(NC)
  [NR] -> TEEM Power/5(NR)
  [NS] -> TEEM Power/4(NS)
  [PwrXDecel_TEEM] -> TEEM Power/3(PwrXDecel_TEEM)
  [PwrInAccel_TEEM] -> TEEM Power/1(PwrInAccel_TEEM)
  Demux2/4 -> [PwrEMP_TEEM]
  Demux2/3 -> [PwrEMC_TEEM]
  Demux2/2 -> [PwrEMR_TEEM]
  Demux2/1 -> [PwrEMS_TEEM]
  Constant2/1 -> Switch/2
  [PwrEMP_TEEM] -> PwrEMP_TEEM/1
  [PwrEMC_TEEM] -> PwrEMC_TEEM/1
  [PwrEMR_TEEM] -> PwrEMR_TEEM/1
  [PwrEMS_TEEM] -> PwrEMS_TEEM/1
  PwrInX_TEEM/1 -> [PwrXDecel_TEEM]
  NC/1 -> [NC]
  NS/1 -> [NS]
  NR/1 -> [NR]
  PwrInHP_TEEM/1 -> [PwrInAccel_TEEM]
  [Pem_TEEM] -> Switch/1
  Constant1/1 -> Switch/3
  Switch/1 -> Demux2/1
  PwrExLP_TEEM/1 -> [PwrExAccel_TEEM]
  [PwrExAccel_TEEM] -> TEEM Power/2(PwrExAccel_TEEM)
  N1cErrN/1 -> [N1cErrN]
  [N1cErrN] -> TEEM Power/7(N1cErrN)
